simulink model "prueba_cadena"  (Simulink 7.5)
settings: Solver=ode45  StartTime=0.1  StopTime=inf  RelTol=1e-3
undefined symbols (not defined in the file or in its folder): cadena1, eslabon1, eslabon2, eslabon3, RootGround, RootPart
libraries: mblibv1 x12
settings Model: Creator=ARTURO  LastModifiedBy=ARTURO
settings HardwareCC: ProdHWDeviceType=Generic->Unspecified (assume 32-bit Generic)
settings SimMechanicsCC: VisOnUpdateDiagram=on  VisDuringSimulation=on

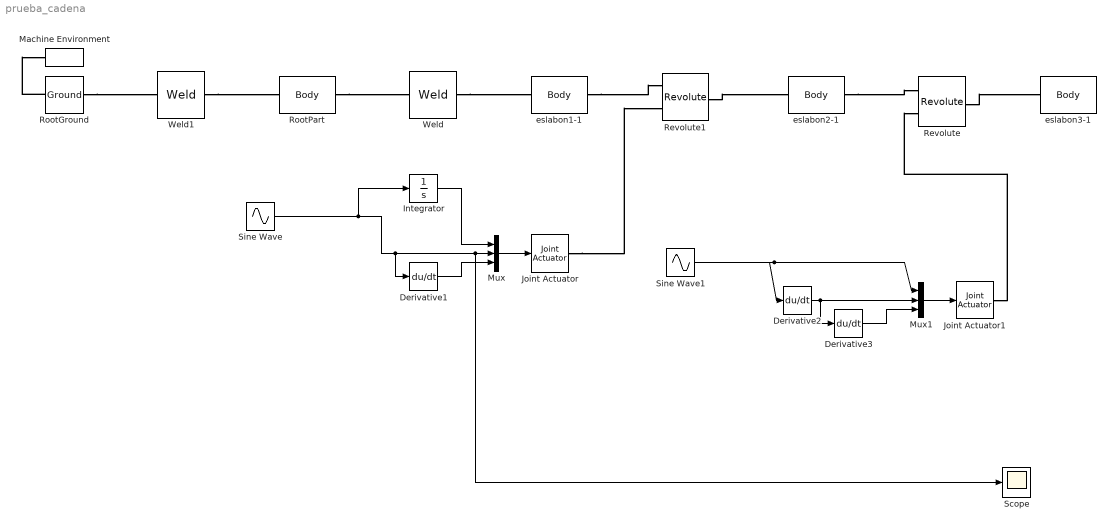
== system prueba_cadena ==
  Derivative1 : Derivative
  Derivative2 : Derivative
  Derivative3 : Derivative
  Integrator : Integrator
  Joint Actuator : mblibv1/Sensors &  Actuators/Joint Actuator  DialogController=MECH.DynMechDlgSource  SystemSampleTime=-1  UpdateFromCAD=off  PhysicalDomain=Mechanical  PortType=blob  ActuationStyle=Motion  AngleUnits=deg  ArcVelocityUnits=deg/s  ArcAccelerationUnits=deg/s^2  CoordPositionUnits=m  VelocityUnits=m/s  AccelerationUnits=m/s^2  ForceUnits=N  TorqueUnits=N*m  ActiveIO=on  Width=3  DialogClass=MechanicalActuatorBlock  Primitive=R1  ReferenceFrame=Absolute (World)
  Joint Actuator1 : mblibv1/Sensors &  Actuators/Joint Actuator  DialogController=MECH.DynMechDlgSource  SystemSampleTime=-1  UpdateFromCAD=off  PhysicalDomain=Mechanical  PortType=blob  ActuationStyle=Motion  AngleUnits=deg  ArcVelocityUnits=deg/s  ArcAccelerationUnits=deg/s^2  CoordPositionUnits=m  VelocityUnits=m/s  AccelerationUnits=m/s^2  ForceUnits=N  TorqueUnits=N*m  ActiveIO=on  Width=3  DialogClass=MechanicalActuatorBlock  Primitive=R1  ReferenceFrame=Absolute (World)
  Machine Environment : mblibv1/Bodies/Machine Environment  DialogController=MECH.DialogSource  SystemSampleTime=-1  PortType=env  PhysicalDomain=Mechanical  DialogTemplateClass=MECH.MachineEnvironment  SyncWhenCopied=off  Gravity=[0 -9.81 0]  GravityUnits=m/s^2  GravityAsSignal=off  Dimensionality=Auto-detect  AnalysisType=Forward dynamics  LinearAssemblyTolerance=1e-3  LinearAssemblyToleranceUnits=m  AngularAssemblyTolerance=1e-3  AngularAssemblyToleranceUnits=rad  ConstraintSolverType=Stabilizing  ConstraintRelTolerance=1e-4  ConstraintAbsTolerance=1e-4  UseRobustSingularityHandling=off  RedundancyAnalysisToleranceType=Automatically select tolerance  RedundancyAnalysisTolerance=1e-14  StatePerturbationType=Fixed  PerturbationSize=1e-5  VisualizeMachine=on  BodyVisualizationType=Use model default body geometries  BodyColorSelMode=Use model default  DefaultBodyColor=[1 0 0]
  Mux : Mux  Inputs=3
  Mux1 : Mux  Inputs=3
  Revolute : mblibv1/Joints/Revolute  DialogController=MECH.DynMechDlgSource  PhysicalDomain=mechanical  SubClassName=Unknown  LeftPortType=blob  RightPortType=blob  LConnTagsString=__newl0|SA1  RConnTagsString=__newr0  UpdateFromCAD=on  PMImportedID=eslabon2-1:-:eslabon3-1  NumSAPorts=1  CutJoint=off  MarkAsCut=off  Primitives=prismatic  PrimitiveProps=R1$World$[0,0,-1]$revolute  DialogClass=JointBlock  R1Axis=[0,0,-1]
  Revolute1 : mblibv1/Joints/Revolute  DialogController=MECH.DynMechDlgSource  PhysicalDomain=mechanical  SubClassName=Unknown  LeftPortType=blob  RightPortType=blob  LConnTagsString=__newl0|SA1  RConnTagsString=__newr0  UpdateFromCAD=on  PMImportedID=eslabon1-1:-:eslabon2-1  NumSAPorts=1  CutJoint=off  MarkAsCut=off  Primitives=prismatic  PrimitiveProps=R1$World$[0,0,1]$revolute  DialogClass=JointBlock  R1Axis=[0,0,1]
  RootGround : mblibv1/Bodies/Ground  DialogController=MECH.DynMechDlgSource  SystemSampleTime=-1  UpdateFromCAD=on  PMImportedID=RootGround  LeftPortType=env  RightPortType=workingframe  PhysicalDomain=Mechanical  DialogClass=GroundBlock  CoordPosition=[0.108201,0.0961923,-0.005]  CoordPositionUnits=m  StateVectorMgrId=0  MachineId=[1 0]  ShowEnvPort=on
  RootPart : mblibv1/Bodies/Body  DialogController=MECH.DynMechDlgSource  PhysicalDomain=mechanical  SubClassName=Unknown  LeftPortType=workingframe  RightPortType=workingframe  LConnTagsString=CS3  RConnTagsString=CS2  UpdateFromCAD=on  PMImportedID=cadena1/RootPart  DialogClass=MechanicalBodyBlock  Mass=0  MassUnits=kg  InertiaUnits=kg*m^2  Inertia=[0,0,0;0,0,0;0,0,0]  Shape=Cylinder  ShapeDims=[1 1]  ShapeUnits=m  ShapeUse=false  Density=1  DensityUnits=kg/m^3  DensityUse=false  GraphicsMode=MACHINE_DEFAULT  BodyColorSelMode=MACHINE_DEFAULT  BodyColor=[1;0;0]  AttachedToCS=CS1  CG=Right$CG$[0.108201 0.0961923 -0.005]$WORLD$WORLD$m$[1 0 0;0 1 0;0 0 1]$3x3 Transform$rad$WORLD$false$cadena1/RootPart::CG(AUTOGEN)  WorkingFrames=Right$CS1$[0 0 0]$WORLD$WORLD$m$[1 0 0;0 1 0;0 0 1]$3x3 Transform$rad$WORLD$false$cadena1/RootPart::CS1(AUTOGEN)#Right$CS2$[-0.0147907 0.0138139 0]$WORLD$WORLD$m$[1 0 0;0 1 0;0 0 1]$3x3 Transform$rad$WORLD$true$cadena1/RootPart:-:eslabon1-1::cadena1/RootPart(AUTOGEN)#Left$CS3$[0.108201 0.0961923 -0.005]$WORLD$WORLD$m$[1 0 0;0 1 0;0 0 1]$3x3 Transform$rad$WORLD$true$RootGround:-:cadena1/RootPart::cadena1/RootPart(AUTOGEN)  CGPos=[0.108201 0.0961923 -0.005]  CGRot=[1 0 0;0 1 0;0 0 1]  CS0Pos=[]  CS0Rot=[]  CS1Pos=[0 0 0]  CS1Rot=[1 0 0;0 1 0;0 0 1]  CS2Pos=[-0.0147907 0.0138139 0]  CS2Rot=[1 0 0;0 1 0;0 0 1]  CS3Pos=[0.108201 0.0961923 -0.005]  CS3Rot=[1 0 0;0 1 0;0 0 1]  CS4Pos=[]  CS4Rot=[]  CS5Pos=[]  CS5Rot=[]  CS6Pos=[]  CS6Rot=[]  CS7Pos=[]  CS7Rot=[]  CS8Pos=[]  CS8Rot=[]  CS9Pos=[]  CS9Rot=[]  CS10Pos=[]  CS10Rot=[]  CS11Pos=[]  CS11Rot=[]  CS12Pos=[]  CS12Rot=[]  CS13Pos=[]  CS13Rot=[]  CS14Pos=[]  CS14Rot=[]  CS15Pos=[]  CS15Rot=[]  CS16Pos=[]  CS16Rot=[]  CS17Pos=[]  CS17Rot=[]  CS18Pos=[]  CS18Rot=[]  CS19Pos=[]  CS19Rot=[]  CS20Pos=[]  CS20Rot=[]
  Scope : Scope
      settings: YMin=4  YMax=7
  Sine Wave : Sin  Amplitude=0  Bias=4  Frequency=0  Phase=0  Samples=10  SampleTime=0  Offset=0
  Sine Wave1 : Sin  Amplitude=22  Bias=0  Frequency=1  Phase=1  Samples=10  SampleTime=0  Offset=0
  Weld : mblibv1/Joints/Weld  DialogController=MECH.DynMechDlgSource  PhysicalDomain=mechanical  SubClassName=Unknown  LeftPortType=blob  RightPortType=blob  LConnTagsString=__newl0  RConnTagsString=__newr0  UpdateFromCAD=on  PMImportedID=cadena1/RootPart:-:eslabon1-1  NumSAPorts=0  CutJoint=off  MarkAsCut=off  Primitives=weld  PrimitiveProps=W$WORLD$[0.57735,0.57735,0.57735]$weld  DialogClass=JointBlock  WAxis=[0.57735,0.57735,0.57735]
  Weld1 : mblibv1/Joints/Weld  DialogController=MECH.DynMechDlgSource  PhysicalDomain=mechanical  SubClassName=Unknown  LeftPortType=blob  RightPortType=blob  LConnTagsString=__newl0  RConnTagsString=__newr0  UpdateFromCAD=on  PMImportedID=RootGround:-:cadena1/RootPart  NumSAPorts=0  CutJoint=off  MarkAsCut=off  Primitives=weld  PrimitiveProps=W$WORLD$[0.57735,0.57735,0.57735]$weld  DialogClass=JointBlock  WAxis=[0.57735,0.57735,0.57735]
  eslabon1-1 : mblibv1/Bodies/Body  DialogController=MECH.DynMechDlgSource  PhysicalDomain=mechanical  SubClassName=Unknown  LeftPortType=workingframe  RightPortType=workingframe  LConnTagsString=CS2  RConnTagsString=CS3  UpdateFromCAD=on  PMImportedID=eslabon1-1  DialogClass=MechanicalBodyBlock  Mass=0.0360868  MassUnits=kg  InertiaUnits=kg*m^2  Inertia=[1.80336e-005,-3.28918e-005,0;-3.28918e-005,8.58612e-005,0;0,0,0.000103744]  Shape=Cylinder  ShapeDims=[1 1]  ShapeUnits=m  ShapeUse=false  Density=1  DensityUnits=kg/m^3  DensityUse=false  GraphicsMode=GFXFILE  GraphicsFileName=cadena1 - eslabon1-1.STL  BodyColorSelMode=COLORPALETTE  BodyColor=[0 0 1]  AttachedToCS=CS1  CG=Right$CG$[-0.0147907 0.0138139 0]$WORLD$WORLD$m$[1 0 0;0 1 0;0 0 1]$3x3 Transform$rad$WORLD$false$eslabon1-1::CG(AUTOGEN)  WorkingFrames=Right$CS1$[-0.00782911 0.019021 -0.0025]$WORLD$WORLD$m$[1 0 0;0 1 0;0 0 1]$3x3 Transform$rad$WORLD$false$eslabon1-1::CS1(AUTOGEN)#Left$CS2$[-0.0147907 0.0138139 0]$WORLD$WORLD$m$[1 0 0;0 1 0;0 0 1]$3x3 Transform$rad$WORLD$true$cadena1/RootPart:-:eslabon1-1::eslabon1-1(AUTOGEN)#Right$CS3$[0.0547178 0.0419844 -0.0025]$WORLD$WORLD$m$[1 0 0;0 1 0;0 0 1]$3x3 Transform$rad$WORLD$true$eslabon1-1:-:eslabon2-1::eslabon1-1(AUTOGEN)  CGPos=[-0.0147907 0.0138139 0]  CGRot=[1 0 0;0 1 0;0 0 1]  CS0Pos=[]  CS0Rot=[]  CS1Pos=[-0.00782911 0.019021 -0.0025]  CS1Rot=[1 0 0;0 1 0;0 0 1]  CS2Pos=[-0.0147907 0.0138139 0]  CS2Rot=[1 0 0;0 1 0;0 0 1]  CS3Pos=[0.0547178 0.0419844 -0.0025]  CS3Rot=[1 0 0;0 1 0;0 0 1]  CS4Pos=[]  CS4Rot=[]  CS5Pos=[]  CS5Rot=[]  CS6Pos=[]  CS6Rot=[]  CS7Pos=[]  CS7Rot=[]  CS8Pos=[]  CS8Rot=[]  CS9Pos=[]  CS9Rot=[]  CS10Pos=[]  CS10Rot=[]  CS11Pos=[]  CS11Rot=[]  CS12Pos=[]  CS12Rot=[]  CS13Pos=[]  CS13Rot=[]  CS14Pos=[]  CS14Rot=[]  CS15Pos=[]  CS15Rot=[]  CS16Pos=[]  CS16Rot=[]  CS17Pos=[]  CS17Rot=[]  CS18Pos=[]  CS18Rot=[]  CS19Pos=[]  CS19Rot=[]  CS20Pos=[]  CS20Rot=[]
  eslabon2-1 : mblibv1/Bodies/Body  DialogController=MECH.DynMechDlgSource  PhysicalDomain=mechanical  SubClassName=Unknown  LeftPortType=workingframe  RightPortType=workingframe  LConnTagsString=CS3  RConnTagsString=CS2  UpdateFromCAD=on  PMImportedID=eslabon2-1  DialogClass=MechanicalBodyBlock  Mass=0.0360868  MassUnits=kg  InertiaUnits=kg*m^2  Inertia=[1.80336e-005,-3.28918e-005,0;-3.28918e-005,8.58612e-005,0;0,0,0.000103744]  Shape=Cylinder  ShapeDims=[1 1]  ShapeUnits=m  ShapeUse=false  Density=1  DensityUnits=kg/m^3  DensityUse=false  GraphicsMode=GFXFILE  GraphicsFileName=cadena1 - eslabon2-1.STL  BodyColorSelMode=COLORPALETTE  BodyColor=[0;0.752941;0]  AttachedToCS=CS1  CG=Right$CG$[0.109898 0.0927796 -0.005]$WORLD$WORLD$m$[0.936251 -0.351332 0;0.351332 0.936251 0;0 0 1]$3x3 Transform$rad$WORLD$false$eslabon2-1::CG(AUTOGEN)  WorkingFrames=Right$CS1$[0.114586 0.1001 -0.0075]$WORLD$WORLD$m$[0.936251 -0.351332 0;0.351332 0.936251 0;0 0 1]$3x3 Transform$rad$WORLD$false$eslabon2-1::CS1(AUTOGEN)#Right$CS2$[0.165078 0.143575 -0.0075]$WORLD$WORLD$m$[1 0 0;0 1 0;0 0 1]$3x3 Transform$rad$WORLD$true$eslabon2-1:-:eslabon3-1::eslabon2-1(AUTOGEN)#Left$CS3$[0.0547178 0.0419844 -0.0025]$WORLD$WORLD$m$[1 0 0;0 1 0;0 0 1]$3x3 Transform$rad$WORLD$true$eslabon1-1:-:eslabon2-1::eslabon2-1(AUTOGEN)  CGPos=[0.109898 0.0927796 -0.005]  CGRot=[0.936251 -0.351332 0;0.351332 0.936251 0;0 0 1]  CS0Pos=[]  CS0Rot=[]  CS1Pos=[0.114586 0.1001 -0.0075]  CS1Rot=[0.936251 -0.351332 0;0.351332 0.936251 0;0 0 1]  CS2Pos=[0.165078 0.143575 -0.0075]  CS2Rot=[1 0 0;0 1 0;0 0 1]  CS3Pos=[0.0547178 0.0419844 -0.0025]  CS3Rot=[1 0 0;0 1 0;0 0 1]  CS4Pos=[]  CS4Rot=[]  CS5Pos=[]  CS5Rot=[]  CS6Pos=[]  CS6Rot=[]  CS7Pos=[]  CS7Rot=[]  CS8Pos=[]  CS8Rot=[]  CS9Pos=[]  CS9Rot=[]  CS10Pos=[]  CS10Rot=[]  CS11Pos=[]  CS11Rot=[]  CS12Pos=[]  CS12Rot=[]  CS13Pos=[]  CS13Rot=[]  CS14Pos=[]  CS14Rot=[]  CS15Pos=[]  CS15Rot=[]  CS16Pos=[]  CS16Rot=[]  CS17Pos=[]  CS17Rot=[]  CS18Pos=[]  CS18Rot=[]  CS19Pos=[]  CS19Rot=[]  CS20Pos=[]  CS20Rot=[]
  eslabon3-1 : mblibv1/Bodies/Body  DialogController=MECH.DynMechDlgSource  PhysicalDomain=mechanical  SubClassName=Unknown  LeftPortType=workingframe  RightPortType=workingframe  LConnTagsString=CS2  UpdateFromCAD=on  PMImportedID=eslabon3-1  DialogClass=MechanicalBodyBlock  Mass=0.0360868  MassUnits=kg  InertiaUnits=kg*m^2  Inertia=[1.80336e-005,-3.28918e-005,0;-3.28918e-005,8.58612e-005,0;0,0,0.000103744]  Shape=Cylinder  ShapeDims=[1 1]  ShapeUnits=m  ShapeUse=false  Density=1  DensityUnits=kg/m^3  DensityUse=false  GraphicsMode=GFXFILE  GraphicsFileName=cadena1 - eslabon3-1.STL  BodyColorSelMode=COLORPALETTE  BodyColor=[1;0;0]  AttachedToCS=CS1  CG=Right$CG$[0.229497 0.181983 -0.01]$WORLD$WORLD$m$[0.98838 -0.152001 0;0.152001 0.98838 0;0 0 1]$3x3 Transform$rad$WORLD$false$eslabon3-1::CG(AUTOGEN)  WorkingFrames=Right$CS1$[0.235586 0.188188 -0.0125]$WORLD$WORLD$m$[0.98838 -0.152001 0;0.152001 0.98838 0;0 0 1]$3x3 Transform$rad$WORLD$false$eslabon3-1::CS1(AUTOGEN)#Left$CS2$[0.165078 0.143575 -0.0075]$WORLD$WORLD$m$[1 0 0;0 1 0;0 0 1]$3x3 Transform$rad$WORLD$true$eslabon2-1:-:eslabon3-1::eslabon3-1(AUTOGEN)  CGPos=[0.229497 0.181983 -0.01]  CGRot=[0.98838 -0.152001 0;0.152001 0.98838 0;0 0 1]  CS0Pos=[]  CS0Rot=[]  CS1Pos=[0.235586 0.188188 -0.0125]  CS1Rot=[0.98838 -0.152001 0;0.152001 0.98838 0;0 0 1]  CS2Pos=[0.165078 0.143575 -0.0075]  CS2Rot=[1 0 0;0 1 0;0 0 1]  CS3Pos=[]  CS3Rot=[]  CS4Pos=[]  CS4Rot=[]  CS5Pos=[]  CS5Rot=[]  CS6Pos=[]  CS6Rot=[]  CS7Pos=[]  CS7Rot=[]  CS8Pos=[]  CS8Rot=[]  CS9Pos=[]  CS9Rot=[]  CS10Pos=[]  CS10Rot=[]  CS11Pos=[]  CS11Rot=[]  CS12Pos=[]  CS12Rot=[]  CS13Pos=[]  CS13Rot=[]  CS14Pos=[]  CS14Rot=[]  CS15Pos=[]  CS15Rot=[]  CS16Pos=[]  CS16Rot=[]  CS17Pos=[]  CS17Rot=[]  CS18Pos=[]  CS18Rot=[]  CS19Pos=[]  CS19Rot=[]  CS20Pos=[]  CS20Rot=[]
  wires:
  Mux/1 -> Joint Actuator/1
  Derivative1/1 -> Mux/3
  Sine Wave1/1 -> Mux1/1, Derivative2/1
  Mux1/1 -> Joint Actuator1/1
  Derivative2/1 -> Mux1/2, Derivative3/1
  Derivative3/1 -> Mux1/3
  Sine Wave/1 -> Derivative1/1, Mux/2, Scope/1, Integrator/1
  Integrator/1 -> Mux/1
  connections:
  RootPart/RConn1 -- Weld/LConn1
  Weld/RConn1 -- eslabon1-1/LConn1
  eslabon2-1/RConn1 -- Revolute/LConn1
  Revolute/RConn1 -- eslabon3-1/LConn1
  eslabon1-1/RConn1 -- Revolute1/LConn1
  Revolute1/RConn1 -- eslabon2-1/LConn1
  RootGround/RConn1 -- Weld1/LConn1
  Weld1/RConn1 -- RootPart/LConn1
  RootGround/LConn1 -- Machine Environment/RConn1
  Joint Actuator/RConn1 -- Revolute1/LConn2
  Joint Actuator1/RConn1 -- Revolute/LConn2
